simulink model "sampleModel330"  (R2021b)
settings: Solver=VariableStepAuto  StartTime=0.0  StopTime=10.0  RelTol=1e-3
libraries: simulink x3
settings Model: Creator=user  LastModifiedBy=user

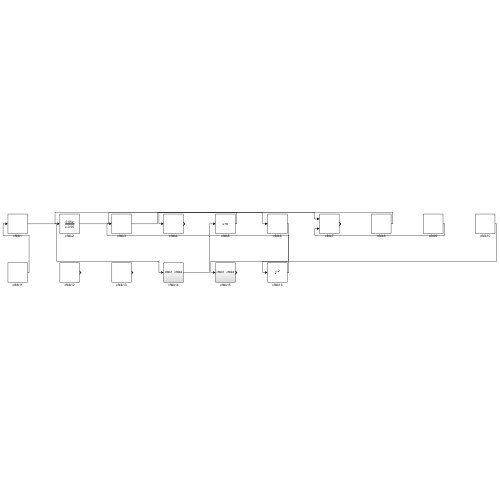
[thumbnail: Simulink's stored preview of the top-level diagram]
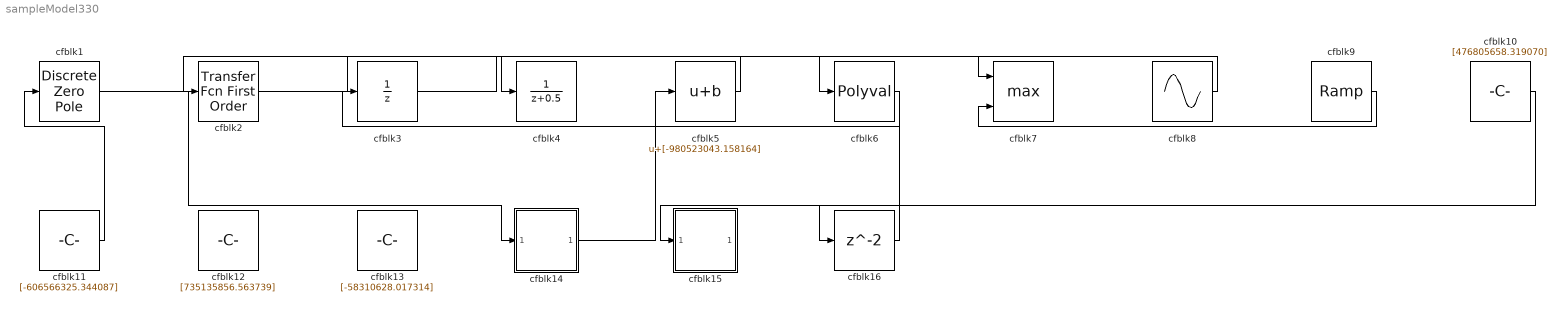
== system sampleModel330 ==
  cfblk1 : DiscreteZeroPole  Poles=[0 0.5]  Gain=1
  cfblk10 : Constant  Value=[476805658.319070]  SampleTime=1
  cfblk11 : Constant  Value=[-606566325.344087]  SampleTime=1
  cfblk12 : Constant  Value=[735135856.563739]  SampleTime=1
  cfblk13 : Constant  Value=[-58310628.017314]  SampleTime=1
  cfblk14 : Subsystem
  cfblk15 : Subsystem
  cfblk16 : Delay  SampleTime=1
  cfblk2 : simulink/Discrete/Transfer Fcn First Order  PoleZ=0.95  ICPrevOutput=0.0  DoSatur=off
  cfblk3 : UnitDelay  HasFrameUpgradeWarning=on
  cfblk4 : DiscreteTransferFcn  SampleTime=1
  cfblk5 : Bias  Bias=[-980523043.158164]
  cfblk6 : Polyval  Coefs=[ +2.081618890e-019, -1.441693666e-014, +4.719686976e-010, -8.536869453e-006, +1.621573104e-001, -8.087801117e+001 ]
  cfblk7 : MinMax  Function=max  Inputs=2
  cfblk8 : Sin  Amplitude=[266263950.415483]  Bias=[584142929.392457]  SampleTime=0
  cfblk9 : simulink/Sources/Ramp  slope=[4745.277346]  start=[6.233419]  InitialOutput=[645142.211114]
  wires:
  cfblk2/1 -> cfblk7/1
  cfblk11/1 -> cfblk1/1
  cfblk1/1 -> cfblk14/1(cfblk1)
  cfblk9/1 -> cfblk7/2
  cfblk5/1 -> cfblk2/1
  cfblk8/1 -> cfblk4/1
  cfblk3/1 -> cfblk6/1
  cfblk10/1 -> cfblk15/1(cfblk1)
  cfblk14/1(cfblk2) -> cfblk5/1
  cfblk6/1 -> cfblk16/1
  cfblk16/1 -> cfblk3/1

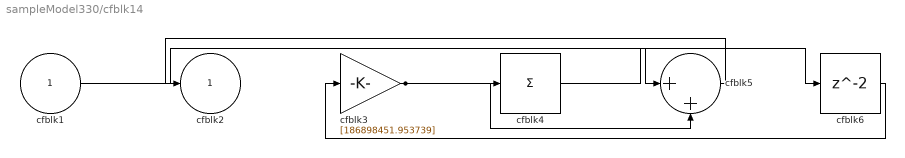
== system sampleModel330/cfblk14 ==
  cfblk1 : Inport
  cfblk3 : Gain  Gain=[186898451.953739]
  cfblk4 : Sum  Inputs=+
  cfblk5 : Sum  Inputs=|++
  cfblk6 : Delay  SampleTime=1
  cfblk2 : Outport
  wires:
  cfblk1/1 -> cfblk5/1
  cfblk3/1 -> cfblk5/2, cfblk4/1
  cfblk5/1 -> cfblk2/1
  cfblk4/1 -> cfblk6/1
  cfblk6/1 -> cfblk3/1

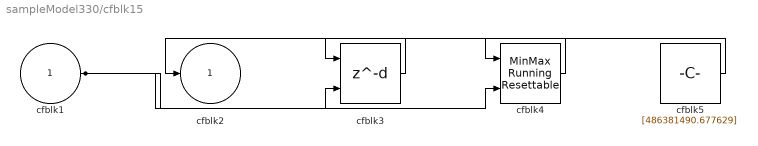
== system sampleModel330/cfblk15 ==
  cfblk1 : Inport
  cfblk3 : Delay  DelayLengthSource=Input port  SampleTime=1
      settings: InputPortMap=u0,p1
  cfblk4 : simulink/Math Operations/MinMax Running Resettable  Function=min  vinit=0.0
  cfblk5 : Constant  Value=[486381490.677629]  SampleTime=1
  cfblk2 : Outport
  wires:
  cfblk5/1 -> cfblk4/1
  cfblk3/1 -> cfblk2/1
  cfblk1/1 -> cfblk4/2, cfblk3/2
  cfblk4/1 -> cfblk3/1
